simulink model "trajectory_controller"  (R2019b)
settings: Solver=VariableStepAuto  StartTime=0.0  StopTime=10.0  RelTol=1e-3
settings Model: Creator=logan  LastModifiedBy=logan

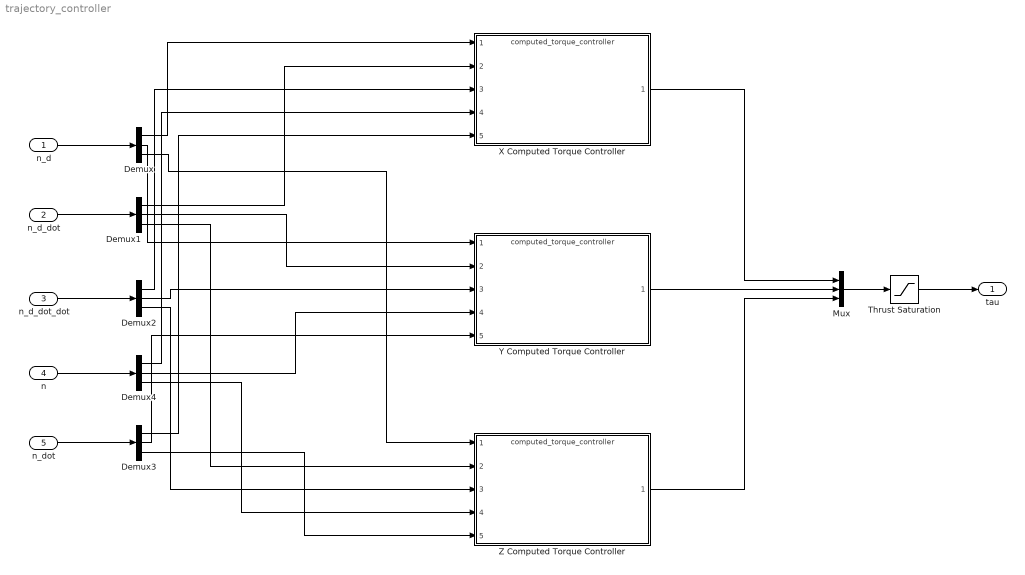
== system trajectory_controller ==
  "n_d " : Inport
  n_d_dot : Inport  Port=2
  n_d_dot_dot : Inport  Port=3
  n : Inport  Port=4
  n_dot : Inport  Port=5
  Demux{,1..4} (5 alike) : Demux  Outputs=3
  Mux : Mux  Inputs=3
  Thrust Saturation : Saturate  UpperLimit=100  LowerLimit=-100
  X Computed Torque Controller : ModelReference  ModelNameDialog=computed_torque_controller.slx  SimulationMode=Normal  ModelReferenceVersion=1.13
  Y Computed Torque Controller : ModelReference  ModelNameDialog=computed_torque_controller.slx  SimulationMode=Normal  ModelReferenceVersion=1.13
  Z Computed Torque Controller : ModelReference  ModelNameDialog=computed_torque_controller.slx  SimulationMode=Normal  ModelReferenceVersion=1.13
  tau : Outport
  wires:
  "n_d "/1 -> Demux/1
  n_d_dot/1 -> Demux1/1
  n_d_dot_dot/1 -> Demux2/1
  Demux/1 -> X Computed Torque Controller/1
  Demux/2 -> Y Computed Torque Controller/1
  Demux/3 -> Z Computed Torque Controller/1
  Demux1/1 -> X Computed Torque Controller/2
  Demux1/2 -> Y Computed Torque Controller/2
  Demux1/3 -> Z Computed Torque Controller/2
  Demux2/1 -> X Computed Torque Controller/3
  Demux2/2 -> Y Computed Torque Controller/3
  Demux2/3 -> Z Computed Torque Controller/3
  n_dot/1 -> Demux3/1
  n/1 -> Demux4/1
  Demux4/1 -> X Computed Torque Controller/4
  Demux4/2 -> Y Computed Torque Controller/4
  Demux3/1 -> X Computed Torque Controller/5
  Demux4/3 -> Z Computed Torque Controller/4
  Demux3/2 -> Y Computed Torque Controller/5
  Demux3/3 -> Z Computed Torque Controller/5
  X Computed Torque Controller/1 -> Mux/1
  Y Computed Torque Controller/1 -> Mux/2
  Z Computed Torque Controller/1 -> Mux/3
  Mux/1 -> Thrust Saturation/1
  Thrust Saturation/1 -> tau/1
